simulink model "Doble_Pendulo_LQR"  (R2023b)
settings: Solver=ode45  StartTime=0.0  StopTime=37  MaxStep=0.001  RelTol=1e-3
values from neighbouring files (symbols this model uses):
  K = lqr(A, B, Q, R)    [Doble_Pendulo.m]
settings Model: Creator=Usuario  LastModifiedBy=Usuario
settings SolverCC: ZeroCrossAlgorithm=Adaptive

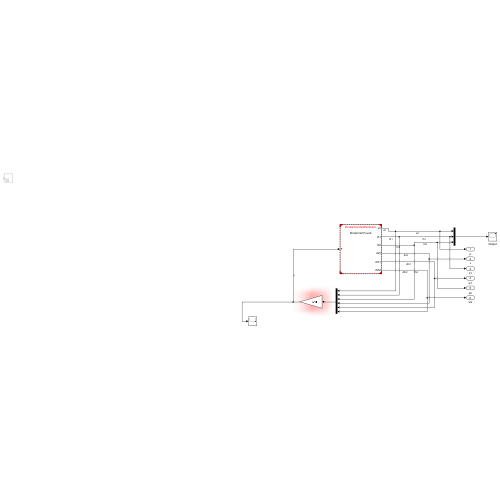
[thumbnail: Simulink's stored preview of the top-level diagram]
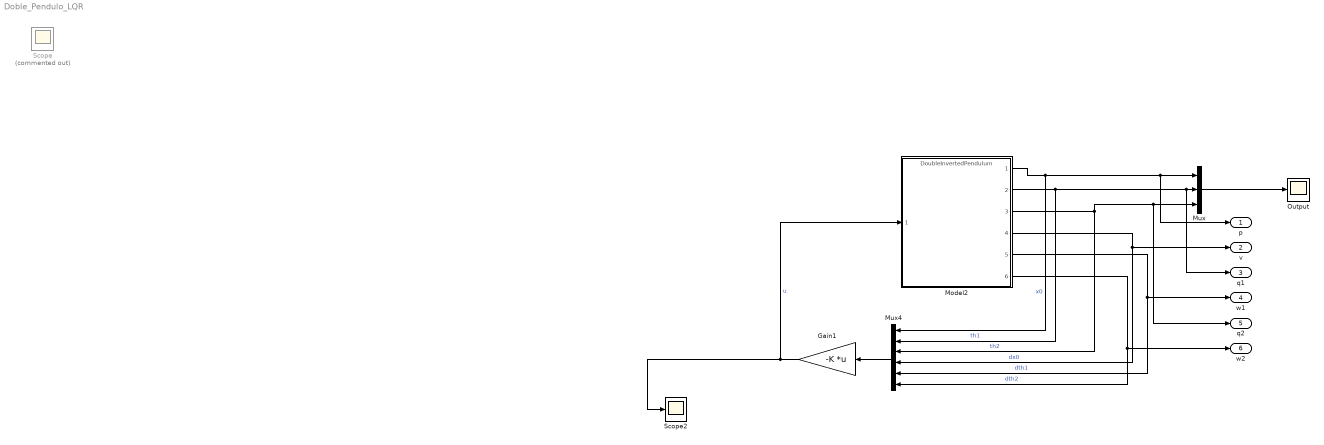
== system Doble_Pendulo_LQR ==
  Gain1 : Gain  Gain=-K  Multiplication=Matrix(K*u)
  Model2 : ModelReference  ModelNameDialog=DoubleInvertedPendulum  SimulationMode=Normal  ModelReferenceVersion=18.17
  Mux : Mux  Inputs=3
  Mux4 : Mux  Inputs=6
  Output : Scope
  Scope : Scope  Commented=on
  Scope2 : Scope
  p : Outport  VectorParamsAs1DForOutWhenUnconnected=off
  v : Outport  Port=2  VectorParamsAs1DForOutWhenUnconnected=off
  q1 : Outport  Port=3  VectorParamsAs1DForOutWhenUnconnected=off
  w1 : Outport  Port=4  VectorParamsAs1DForOutWhenUnconnected=off
  q2 : Outport  Port=5  VectorParamsAs1DForOutWhenUnconnected=off
  w2 : Outport  Port=6  VectorParamsAs1DForOutWhenUnconnected=off
  wires:
  Model2/6 -> Mux4/6, w2/1  "dth2"
  Model2/2 -> q1/1, Mux/2, Mux4/2  "th1"
  Mux4/1 -> Gain1/1
  Gain1/1 -> Model2/1, Scope2/1  "u"
  Model2/4 -> v/1, Mux4/4  "dx0"
  Model2/3 -> q2/1, Mux/3, Mux4/3  "th2"
  Model2/5 -> w1/1, Mux4/5  "dth1"
  Model2/1 -> p/1, Mux/1, Mux4/1  "x0"
  Mux/1 -> Output/1
